simulink model "InvertedPend"  (R2022b)
settings: Solver=VariableStepAuto  StartTime=0.0  StopTime=100.0  RelTol=1e-3
values from neighbouring files (symbols this model uses):
  A = [0 1; cos(theta(1)) -b/(m*L^2)]    [invPend.m]
  b = 0.01    [invPend.m]
  B = [0 1/(m*L^2)]'    [invPend.m]
  C = [0 1]    [invPend.m]
  g = 9.83    [invPend.m]
  Kr = lqr(sysA, sysB, sysQ, sysR)    [buildLQGInvert.m]
  L = 1    [invPend.m]
  m = 1    [invPend.m]
undefined symbols (not defined in the file or in its folder): Ke
settings Model: Creator=abane  LastModifiedBy=abane

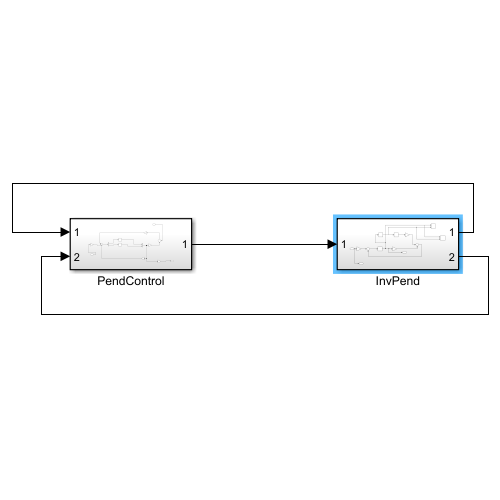
[thumbnail: Simulink's stored preview of the top-level diagram]
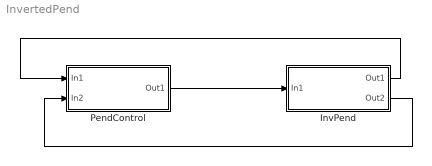
== system InvertedPend ==
  InvPend : Subsystem
  PendControl : Subsystem
  wires:
  PendControl/1(Out1) -> InvPend/1(In1)
  InvPend/2(Out2) -> PendControl/2(In2)
  InvPend/1(Out1) -> PendControl/1(In1)

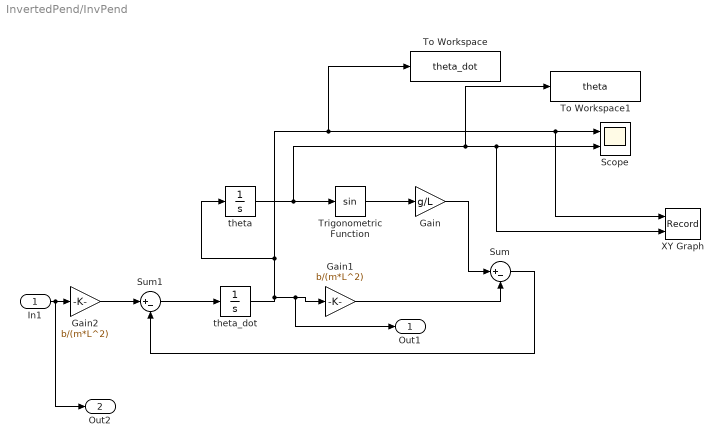
== system InvertedPend/InvPend ==
  In1 : Inport
  Gain : Gain  Gain=g/L
  Gain1 : Gain  Gain=b/(m*L^2)
  Gain2 : Gain  Gain=b/(m*L^2)
  Scope : Scope  NumInputPorts=2
  Sum : Sum  Inputs=|+-
  Sum1 : Sum  Inputs=|+-
  To Workspace : ToWorkspace  VariableName=theta_dot  SaveFormat=Timeseries  SampleTime=-1
  To Workspace1 : ToWorkspace  VariableName=theta  SaveFormat=Timeseries  SampleTime=-1
  Trigonometric Function : Trigonometry  ApproximationMethod=CORDIC
  XY Graph : Record  FileSettingsInternal="{\"entries\":[{\"content\":{\"excelSettings\":{\"content\":{},\"type\":\"Streamout.ExcelSettings\"}},\"type\":\"Streamout.FileSettingStorage\",\"uuid\":\"51e2709a-467c-4936-991f-6ae7cd074600\"}],\"packageUris\":[\"http://schema.mathworks.com/mf0/streamout_blocks/R2020a\"],\"version\":\"1.0\"}"  Layout=[1 1]  SignalsInternal="{\"entries\":[{\"content\":{\"signals\":[{\"content\":{\"blockPath\":[\"InvertedPend/InvPend/XY Graph\"],\"channel\":[],\"dimensions\":[1],\"domain\":\"InvertedPend/InvPend/XY Graph\",\"lineColor\":\"#a2142f\",\"plots\":[1],\"port\":1,\"sid\":[\"\"],\"signalID\":47,\"signalName\":\"theta_dot\"},\"type\":\"RecordBlkView.Signal\",\"uuid\":\"224a0f99-98df-42da-a84f-d3c95a34cb93\"},{\"content\":{\"blockPath\":[\"InvertedPend/InvPend/XY Graph\"],\"channel\":[],\"dimensions\":[1],\"domain\":\"InvertedPend/InvPend/XY Graph\",\"lineColor\":\"#139fff\",\"plots\":[1],\"port\":2,\"sid\":[\"\"],\"signalID\":51,\"signalName\":\"theta\"},\"type\":\"RecordBlkView.Signal\",\"uuid\":\"b560b89e-def1-4323-a5ad-ec560ba504d8\"}]},\"type\":\"RecordBlkView.InputSignals\",\"uuid\":\"2dd17b51-3891-47f4-ad94-c7502cc63b3e\"}],\"packageUris\":[\"http://schema.mathworks.com/mf0/streamout_blocks/R2020a\"],\"version\":\"1.0\"}"  VisualizationBindings="{\"xyplotplugin\":{\"info\":[{\"series\":[{\"bindingParametersList\":[{\"parameter\":\"X-Axis\",\"signalID\":47,\"signalName\":\"theta_dot\"},{\"parameter\":\"Y-Axis\",\"signalID\":51,\"signalName\":\"theta\"}],\"seriesID\":63900}],\"subplotID\":1}]}}"  CompatibilityTag=XY
  theta : Integrator  InitialCondition=-2
  theta_dot : Integrator  InitialCondition=4
  Out1 : Outport
  Out2 : Outport  Port=2
  wires:
  theta_dot/1 -> Out1/1, Gain1/1, To Workspace/1, XY Graph/1, Scope/1, theta/1
  theta/1 -> To Workspace1/1, XY Graph/2, Scope/2, Trigonometric Function/1
  Trigonometric Function/1 -> Gain/1
  Gain1/1 -> Sum/2
  Gain/1 -> Sum/1
  Sum/1 -> Sum1/2
  Gain2/1 -> Sum1/1
  Sum1/1 -> theta_dot/1
  In1/1 -> Out2/1, Gain2/1

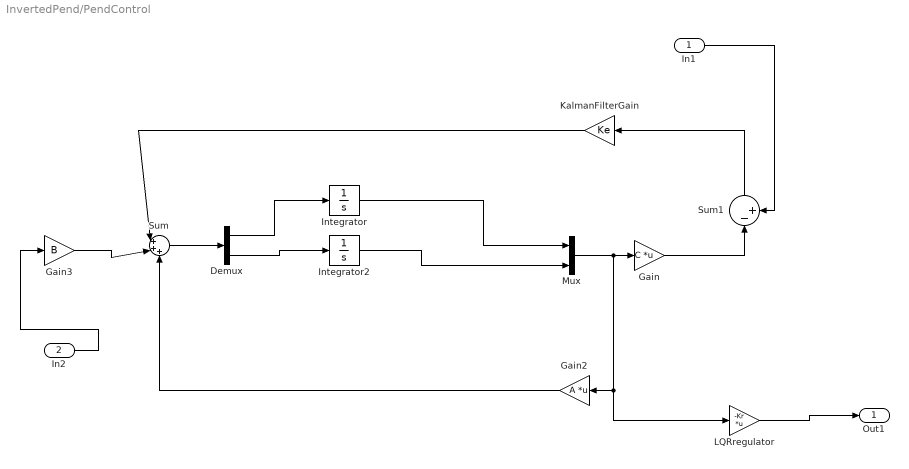
== system InvertedPend/PendControl ==
  In1 : Inport
  In2 : Inport  Port=2
  Demux : Demux  Outputs=2
  Gain : Gain  Gain=C  Multiplication=Matrix(K*u)
  Gain2 : Gain  Gain=A  Multiplication=Matrix(K*u)
  Gain3 : Gain  Gain=B
  Integrator : Integrator
  Integrator2 : Integrator
  KalmanFilterGain : Gain  Gain=Ke
  LQRregulator : Gain  Gain=-Kr  Multiplication=Matrix(K*u)
  Mux : Mux  Inputs=2
  Sum : Sum  Inputs=|+++
  Sum1 : Sum  Inputs=|-+
  Out1 : Outport
  wires:
  Sum/1 -> Demux/1
  Demux/1 -> Integrator/1
  Integrator/1 -> Mux/1
  Mux/1 -> LQRregulator/1, Gain2/1, Gain/1
  Gain/1 -> Sum1/1
  Sum1/1 -> KalmanFilterGain/1
  KalmanFilterGain/1 -> Sum/1
  Gain2/1 -> Sum/3
  Gain3/1 -> Sum/2
  LQRregulator/1 -> Out1/1
  In2/1 -> Gain3/1
  Demux/2 -> Integrator2/1
  Integrator2/1 -> Mux/2
  In1/1 -> Sum1/2
